simulink model "SerieRuidoFiltrado"  (Simulink 7.2)
settings: Solver=ode3  StartTime=Intime  StopTime=Sttime  FixedStep=10^-3  RelTol=1e-3
values from neighbouring files (symbols this model uses):
  FTf = 1/mag*FTfp    [Filtros.m]    (also in RuidoFiltroN.m)
  FTf2 = 1/mag2*FTfp2    [Filtros.m]    (also in RuidoFiltroN.m)
  Intime = 0    [Filtros.m]    (also in RuidoFiltroN.m)
  Sttime = 40    [Filtros.m]    (also in RuidoFiltroN.m = 20)
  tsub = 2    [Filtros.m]    (also in RuidoFiltroN.m)
libraries: simulink x1
settings Model: Creator=Ferdinando  LastModifiedBy=FVOliveira
settings DebuggingCC: StrictBusMsg=ErrorLevel1

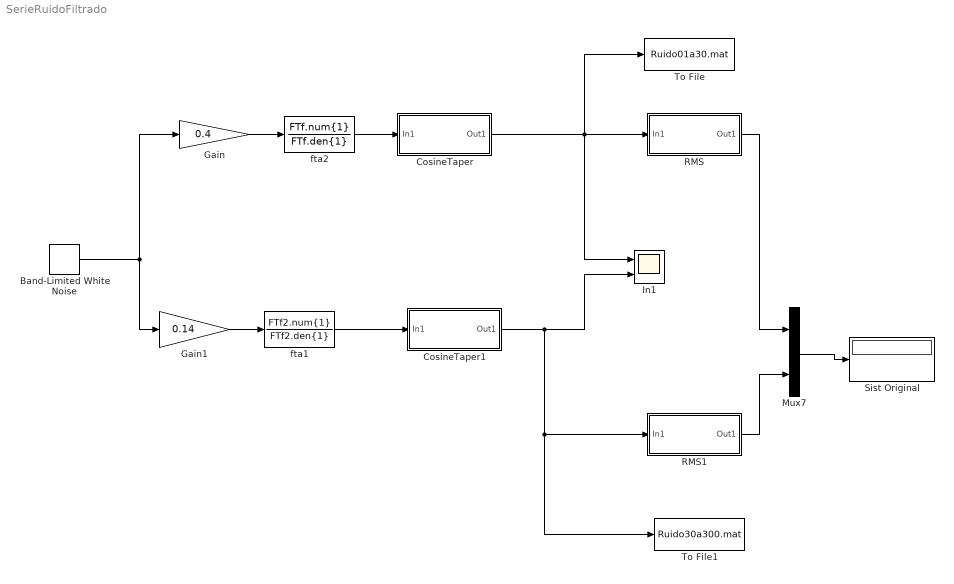
== system SerieRuidoFiltrado ==
  Band-Limited White Noise : simulink/Sources/Band-Limited White Noise  SystemSampleTime=-1  Cov=1  Ts=10^-3  seed=[23341]
  CosineTaper : Subsystem  TreatAsAtomicUnit=on
  CosineTaper1 : Subsystem  TreatAsAtomicUnit=on
  Gain : Gain  Gain=0.4  ParameterDataType=fixdt(1, 16)  ParameterScaling=2^0  OutDataType=fixdt(1, 16)  OutScaling=2^0
  Gain1 : Gain  Gain=0.14  ParameterDataType=fixdt(1, 16)  ParameterScaling=2^0  OutDataType=fixdt(1, 16)  OutScaling=2^0
  In1 : Scope  NumInputPorts=2
      settings: YMin=-5~-5  YMax=5~5  SaveName=Rand3and
  Mux7 : Mux  Inputs=2
  RMS : Subsystem  TreatAsAtomicUnit=on
  RMS1 : Subsystem  TreatAsAtomicUnit=on
  Sist Original : Display
  To File : ToFile  Filename=Ruido01a30.mat  MatrixName=Ruido
  To File1 : ToFile  Filename=Ruido30a300.mat  MatrixName=Ruido
  fta1 : TransferFcn  Numerator=FTf2.num{1}  Denominator=FTf2.den{1}
  fta2 : TransferFcn  Numerator=FTf.num{1}  Denominator=FTf.den{1}
  wires:
  Gain/1 -> fta2/1
  Band-Limited White Noise/1 -> Gain/1, Gain1/1
  RMS/1(Out1) -> Mux7/1
  RMS1/1(Out1) -> Mux7/2
  Mux7/1 -> Sist Original/1
  Gain1/1 -> fta1/1
  fta1/1 -> CosineTaper1/1(In1)
  fta2/1 -> CosineTaper/1(In1)
  CosineTaper/1(Out1) -> In1/1, RMS/1(In1), To File/1
  CosineTaper1/1(Out1) -> In1/2, RMS1/1(In1), To File1/1

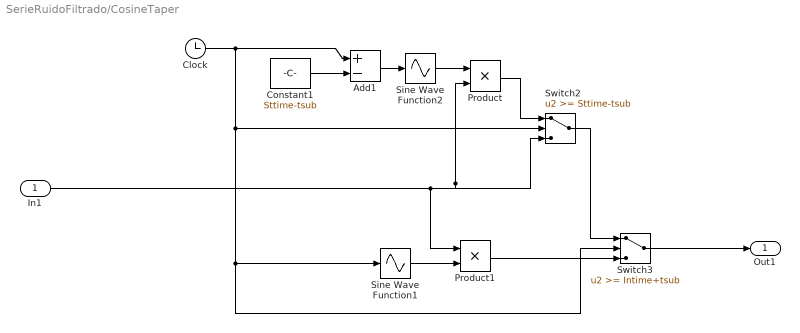
== system SerieRuidoFiltrado/CosineTaper ==
  In1 : Inport  OutDataType=sfix(16)  OutScaling=2^0
  Add1 : Sum  Inputs=+-  OutDataType=sfix(16)  OutScaling=2^-10
  Clock : Clock
      settings: Decimation=10
  Constant1 : Constant  Value=Sttime-tsub  OutDataType=sfix(16)  OutScaling=2^0
  Product : Product  OutDataType=sfix(16)  OutScaling=2^0  RndMeth=Zero
  Product1 : Product  OutDataType=sfix(16)  OutScaling=2^0  RndMeth=Zero
  Sine Wave Function1 : Sin  TimeSource=Use external signal  Amplitude=0.5  Bias=0.5  Frequency=pi/tsub  Phase=-pi/2  SampleTime=0
  Sine Wave Function2 : Sin  TimeSource=Use external signal  Amplitude=0.5  Bias=0.5  Frequency=pi/tsub  Phase=pi/2  SampleTime=0
  Switch2 : Switch  Threshold=Sttime-tsub  OutDataType=fixdt(1, 16)  OutScaling=2^0
  Switch3 : Switch  Threshold=Intime+tsub  OutDataType=fixdt(1, 16)  OutScaling=2^0
  Out1 : Outport  OutDataType=sfix(16)  OutScaling=2^0
  wires:
  Constant1/1 -> Add1/2
  Add1/1 -> Sine Wave Function2/1
  Sine Wave Function2/1 -> Product/1
  Product/1 -> Switch2/1
  In1/1 -> Product/2, Switch2/3, Product1/1
  Switch2/1 -> Switch3/1
  Clock/1 -> Add1/1, Switch2/2, Sine Wave Function1/1, Switch3/2
  Sine Wave Function1/1 -> Product1/2
  Product1/1 -> Switch3/3
  Switch3/1 -> Out1/1

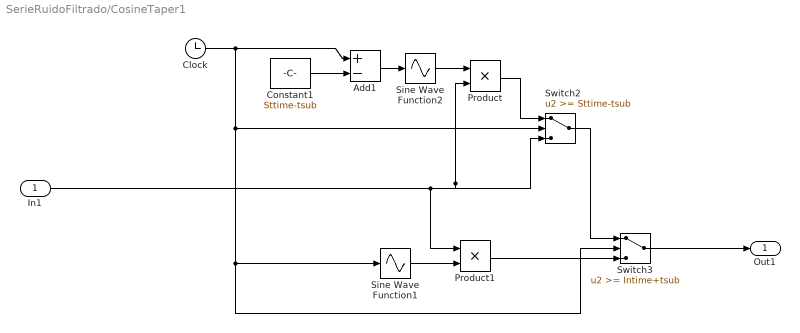
== system SerieRuidoFiltrado/CosineTaper1 ==
  In1 : Inport  OutDataType=sfix(16)  OutScaling=2^0
  Add1 : Sum  Inputs=+-  OutDataType=sfix(16)  OutScaling=2^-10
  Clock : Clock
      settings: Decimation=10
  Constant1 : Constant  Value=Sttime-tsub  OutDataType=sfix(16)  OutScaling=2^0
  Product : Product  OutDataType=sfix(16)  OutScaling=2^0  RndMeth=Zero
  Product1 : Product  OutDataType=sfix(16)  OutScaling=2^0  RndMeth=Zero
  Sine Wave Function1 : Sin  TimeSource=Use external signal  Amplitude=0.5  Bias=0.5  Frequency=pi/tsub  Phase=-pi/2  SampleTime=0
  Sine Wave Function2 : Sin  TimeSource=Use external signal  Amplitude=0.5  Bias=0.5  Frequency=pi/tsub  Phase=pi/2  SampleTime=0
  Switch2 : Switch  Threshold=Sttime-tsub  OutDataType=fixdt(1, 16)  OutScaling=2^0
  Switch3 : Switch  Threshold=Intime+tsub  OutDataType=fixdt(1, 16)  OutScaling=2^0
  Out1 : Outport  OutDataType=sfix(16)  OutScaling=2^0
  wires:
  Constant1/1 -> Add1/2
  Add1/1 -> Sine Wave Function2/1
  Sine Wave Function2/1 -> Product/1
  Product/1 -> Switch2/1
  In1/1 -> Product/2, Switch2/3, Product1/1
  Switch2/1 -> Switch3/1
  Clock/1 -> Add1/1, Switch2/2, Sine Wave Function1/1, Switch3/2
  Sine Wave Function1/1 -> Product1/2
  Product1/1 -> Switch3/3
  Switch3/1 -> Out1/1

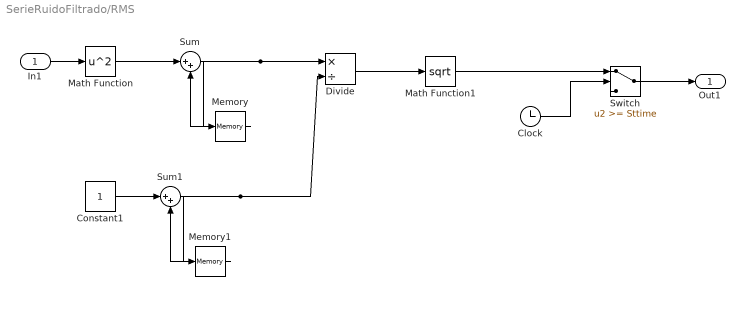
== system SerieRuidoFiltrado/RMS ==
  In1 : Inport  OutDataType=sfix(16)  OutScaling=2^0
  Clock : Clock
      settings: Decimation=10
  Constant1 : Constant  OutDataType=sfix(16)  OutScaling=2^0
  Divide : Product  Inputs=*/  OutDataType=fixdt(1, 16)  OutScaling=2^-10
  Math Function : Math  Operator=square  OutDataType=fixdt(1, 16)  OutScaling=2^0  SaturateOnIntegerOverflow=on
  Math Function1 : Math  Operator=sqrt  OutDataType=sfix(16)  OutScaling=2^0  SaturateOnIntegerOverflow=on
  Memory : Memory  InheritSampleTime=on
  Memory1 : Memory  InheritSampleTime=on
  Sum : Sum  Inputs=|++  OutDataType=sfix(16)  OutScaling=2^0  SaturateOnIntegerOverflow=on  InputSameDT=on  OutDataTypeStr=Inherit: Same as first input
  Sum1 : Sum  Inputs=|++  OutDataType=sfix(16)  OutScaling=2^0  SaturateOnIntegerOverflow=on  InputSameDT=on  OutDataTypeStr=Inherit: Same as first input
  Switch : Switch  Threshold=Sttime  OutDataType=fixdt(1, 16)  OutScaling=2^0
  Out1 : Outport  OutDataType=sfix(16)  OutScaling=2^0
  wires:
  In1/1 -> Math Function/1
  Sum/1 -> Memory/1, Divide/1
  Memory/1 -> Sum/2
  Sum1/1 -> Memory1/1, Divide/2
  Memory1/1 -> Sum1/2
  Constant1/1 -> Sum1/1
  Divide/1 -> Math Function1/1
  Math Function/1 -> Sum/1
  Clock/1 -> Switch/2
  Switch/1 -> Out1/1
  Math Function1/1 -> Switch/1

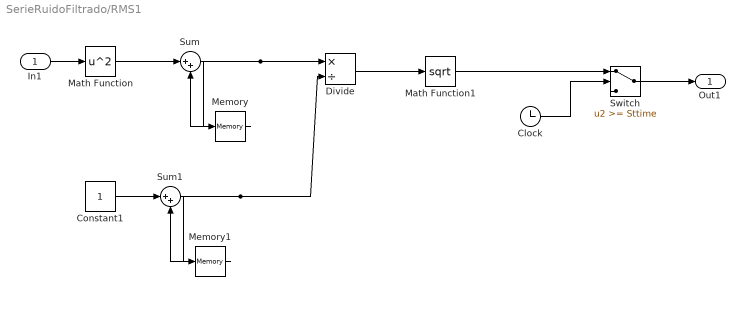
== system SerieRuidoFiltrado/RMS1 ==
  In1 : Inport  OutDataType=sfix(16)  OutScaling=2^0
  Clock : Clock
      settings: Decimation=10
  Constant1 : Constant  OutDataType=sfix(16)  OutScaling=2^0
  Divide : Product  Inputs=*/  OutDataType=fixdt(1, 16)  OutScaling=2^-10
  Math Function : Math  Operator=square  OutDataType=fixdt(1, 16)  OutScaling=2^0  SaturateOnIntegerOverflow=on
  Math Function1 : Math  Operator=sqrt  OutDataType=sfix(16)  OutScaling=2^0  SaturateOnIntegerOverflow=on
  Memory : Memory  InheritSampleTime=on
  Memory1 : Memory  InheritSampleTime=on
  Sum : Sum  Inputs=|++  OutDataType=sfix(16)  OutScaling=2^0  SaturateOnIntegerOverflow=on  InputSameDT=on  OutDataTypeStr=Inherit: Same as first input
  Sum1 : Sum  Inputs=|++  OutDataType=sfix(16)  OutScaling=2^0  SaturateOnIntegerOverflow=on  InputSameDT=on  OutDataTypeStr=Inherit: Same as first input
  Switch : Switch  Threshold=Sttime  OutDataType=fixdt(1, 16)  OutScaling=2^0
  Out1 : Outport  OutDataType=sfix(16)  OutScaling=2^0
  wires:
  In1/1 -> Math Function/1
  Sum/1 -> Memory/1, Divide/1
  Memory/1 -> Sum/2
  Sum1/1 -> Memory1/1, Divide/2
  Memory1/1 -> Sum1/2
  Constant1/1 -> Sum1/1
  Divide/1 -> Math Function1/1
  Math Function/1 -> Sum/1
  Clock/1 -> Switch/2
  Switch/1 -> Out1/1
  Math Function1/1 -> Switch/1
